simulink library "HardwareCommunication"  (R2016b)
settings: Solver=VariableStepAuto  StartTime=0.0  StopTime=10.0  RelTol=1e-3
undefined symbols (not defined in the file or in its folder): ReceiveFromInputDevice, SendToInputDevice
libraries: inSOMANET x8, SendToSOMANET x8, VariousLibrary x4, GESHandler x3, InputDeviceHandler x3, PDBHandler x3, SOMANETHandler x3, xpcethercatlib x2, ReceiveFromGES x2, ReceiveFromPDB x2, SendToPDB x2, InCommunication x1
settings Model: Creator=march  LastModifiedBy=march

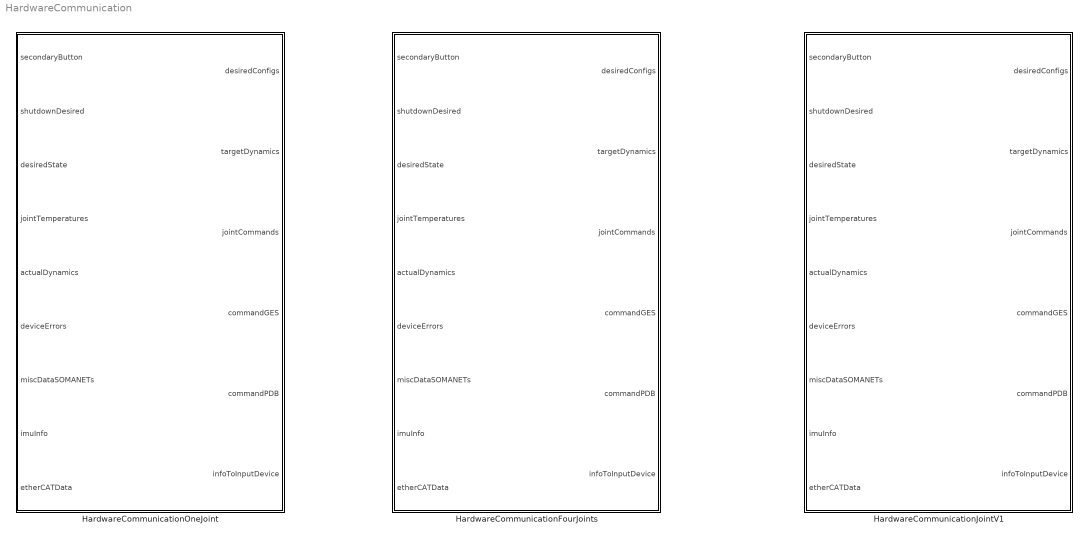
== system HardwareCommunication ==
  HardwareCommunicationFourJoints : Subsystem
  HardwareCommunicationJointV1 : Subsystem  AncestorBlock=HardwareCommunication/HardwareCommunicationOneJoint
  HardwareCommunicationOneJoint : Subsystem

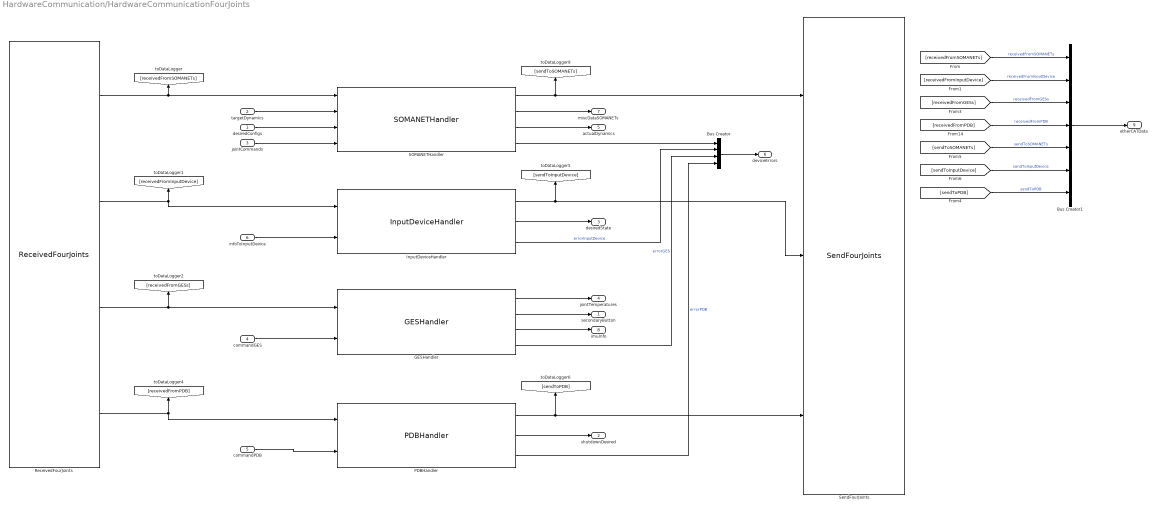
== system HardwareCommunication/HardwareCommunicationFourJoints ==
  desiredConfigs : Inport
  targetDynamics : Inport  Port=2
  jointCommands : Inport  Port=3
  commandGES : Inport  Port=4
  commandPDB : Inport  Port=5
  infoToInputDevice : Inport  Port=6
  Bus Creator : BusCreator  Inputs=4  OutDataTypeStr=Bus: DeviceErrors  NonVirtualBus=on
  Bus Creator1 : BusCreator  Inputs=7  OutDataTypeStr=Bus: EtherCATData  NonVirtualBus=on
  GESHandler : GESHandler/GESHandler
  InputDeviceHandler : InputDeviceHandler/InputDeviceHandler
  PDBHandler : PDBHandler/PDBHandler
  ReceivedFourJoints : InCommunication/ReceivedFourJoints
  SOMANETHandler : SOMANETHandler/SOMANETHandler
  SendFourJoints : OutCommunication/SendFourJoints
  secondaryButton : Outport
  shutdownDesired : Outport  Port=2
  desiredState : Outport  Port=3
  jointTemperatures : Outport  Port=4
  actualDynamics : Outport  Port=5
  deviceErrors : Outport  Port=6
  miscDataSOMANETs : Outport  Port=7
  imuInfo : Outport  Port=8
  etherCATData : Outport  Port=9
  wires:
  infoToInputDevice/1 -> InputDeviceHandler/2
  ReceivedFourJoints/3 -> GESHandler/1, [receivedFromGESs]
  ReceivedFourJoints/2 -> InputDeviceHandler/1, [receivedFromInputDevice]
  ReceivedFourJoints/4 -> PDBHandler/1, [receivedFromPDB]
  InputDeviceHandler/1 -> SendFourJoints/2, [sendToInputDevice]
  InputDeviceHandler/3 -> Bus Creator/2  "errorInputDevice"
  Bus Creator/1 -> deviceErrors/1
  PDBHandler/1 -> SendFourJoints/3, [sendToPDB]
  [receivedFromInputDevice] -> Bus Creator1/2  "receivedFromInputDevice"
  [receivedFromSOMANETs] -> Bus Creator1/1  "receivedFromSOMANETs"
  SOMANETHandler/2 -> miscDataSOMANETs/1
  [sendToPDB] -> Bus Creator1/7  "sendToPDB"
  ReceivedFourJoints/1 -> [receivedFromSOMANETs], SOMANETHandler/1
  GESHandler/2 -> secondaryButton/1
  SOMANETHandler/1 -> SendFourJoints/1, [sendToSOMANETs]
  InputDeviceHandler/2 -> desiredState/1
  jointCommands/1 -> SOMANETHandler/4
  SOMANETHandler/3 -> actualDynamics/1
  [sendToSOMANETs] -> Bus Creator1/5  "sendToSOMANETs"
  [sendToInputDevice] -> Bus Creator1/6  "sendToInputDevice"
  [receivedFromGESs] -> Bus Creator1/3  "receivedFromGESs"
  SOMANETHandler/4 -> Bus Creator/1
  desiredConfigs/1 -> SOMANETHandler/3
  [receivedFromPDB] -> Bus Creator1/4  "receivedFromPDB"
  Bus Creator1/1 -> etherCATData/1
  GESHandler/1 -> jointTemperatures/1
  PDBHandler/3 -> Bus Creator/4  "errorPDB"
  commandGES/1 -> GESHandler/2
  GESHandler/4 -> Bus Creator/3  "errorGES"
  commandPDB/1 -> PDBHandler/2
  PDBHandler/2 -> shutdownDesired/1
  targetDynamics/1 -> SOMANETHandler/2
  GESHandler/3 -> imuInfo/1

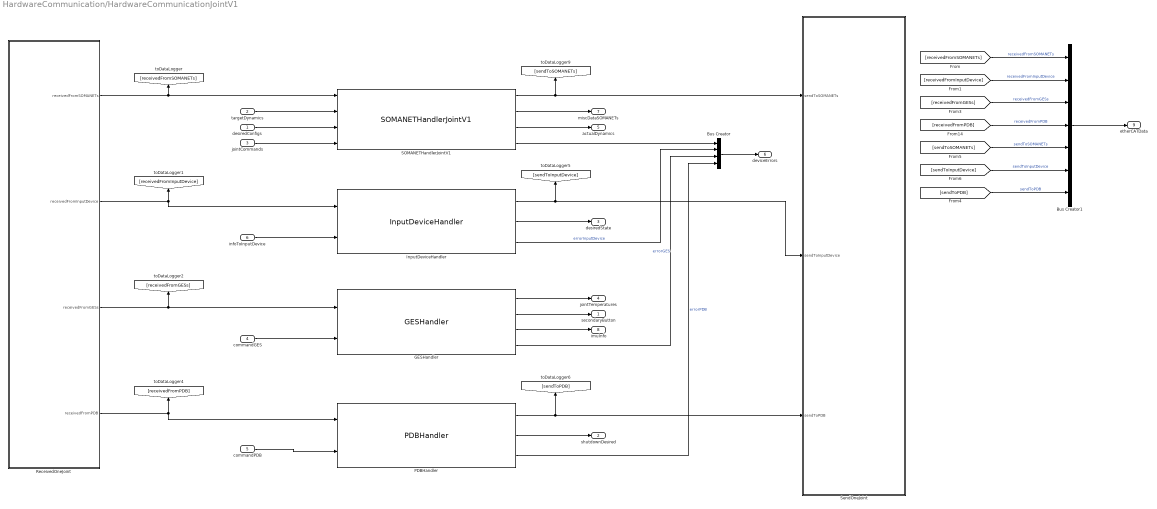
== system HardwareCommunication/HardwareCommunicationJointV1 ==
  desiredConfigs : Inport
  targetDynamics : Inport  Port=2
  jointCommands : Inport  Port=3
  commandGES : Inport  Port=4
  commandPDB : Inport  Port=5
  infoToInputDevice : Inport  Port=6
  Bus Creator : BusCreator  Inputs=4  OutDataTypeStr=Bus: DeviceErrors  NonVirtualBus=on
  Bus Creator1 : BusCreator  Inputs=7  OutDataTypeStr=Bus: EtherCATData  NonVirtualBus=on
  GESHandler : GESHandler/GESHandler
  InputDeviceHandler : InputDeviceHandler/InputDeviceHandler
  PDBHandler : PDBHandler/PDBHandler
  ReceivedOneJoint : Subsystem  AncestorBlock=InCommunication/ReceivedOneJoint
  SOMANETHandlerJointV1 : SOMANETHandler/SOMANETHandlerJointV1
  SendOneJoint : Subsystem  AncestorBlock=OutCommunication/SendOneJoint
  secondaryButton : Outport
  shutdownDesired : Outport  Port=2
  desiredState : Outport  Port=3
  jointTemperatures : Outport  Port=4
  actualDynamics : Outport  Port=5
  deviceErrors : Outport  Port=6
  miscDataSOMANETs : Outport  Port=7
  imuInfo : Outport  Port=8
  etherCATData : Outport  Port=9
  wires:
  infoToInputDevice/1 -> InputDeviceHandler/2
  ReceivedOneJoint/3(receivedFromGESs) -> GESHandler/1, [receivedFromGESs]
  ReceivedOneJoint/2(receivedFromInputDevice) -> InputDeviceHandler/1, [receivedFromInputDevice]
  ReceivedOneJoint/4(receivedFromPDB) -> PDBHandler/1, [receivedFromPDB]
  InputDeviceHandler/1 -> SendOneJoint/2(sendToInputDevice), [sendToInputDevice]
  InputDeviceHandler/3 -> Bus Creator/2  "errorInputDevice"
  Bus Creator/1 -> deviceErrors/1
  PDBHandler/1 -> SendOneJoint/3(sendToPDB), [sendToPDB]
  [receivedFromInputDevice] -> Bus Creator1/2  "receivedFromInputDevice"
  [receivedFromSOMANETs] -> Bus Creator1/1  "receivedFromSOMANETs"
  SOMANETHandlerJointV1/2 -> miscDataSOMANETs/1
  [sendToPDB] -> Bus Creator1/7  "sendToPDB"
  ReceivedOneJoint/1(receivedFromSOMANETs) -> SOMANETHandlerJointV1/1, [receivedFromSOMANETs]
  GESHandler/2 -> secondaryButton/1
  SOMANETHandlerJointV1/1 -> SendOneJoint/1(sendToSOMANETs), [sendToSOMANETs]
  InputDeviceHandler/2 -> desiredState/1
  jointCommands/1 -> SOMANETHandlerJointV1/4
  SOMANETHandlerJointV1/3 -> actualDynamics/1
  [sendToSOMANETs] -> Bus Creator1/5  "sendToSOMANETs"
  [sendToInputDevice] -> Bus Creator1/6  "sendToInputDevice"
  [receivedFromGESs] -> Bus Creator1/3  "receivedFromGESs"
  SOMANETHandlerJointV1/4 -> Bus Creator/1
  desiredConfigs/1 -> SOMANETHandlerJointV1/3
  [receivedFromPDB] -> Bus Creator1/4  "receivedFromPDB"
  Bus Creator1/1 -> etherCATData/1
  GESHandler/1 -> jointTemperatures/1
  PDBHandler/3 -> Bus Creator/4  "errorPDB"
  commandGES/1 -> GESHandler/2
  GESHandler/4 -> Bus Creator/3  "errorGES"
  commandPDB/1 -> PDBHandler/2
  PDBHandler/2 -> shutdownDesired/1
  targetDynamics/1 -> SOMANETHandlerJointV1/2
  GESHandler/3 -> imuInfo/1

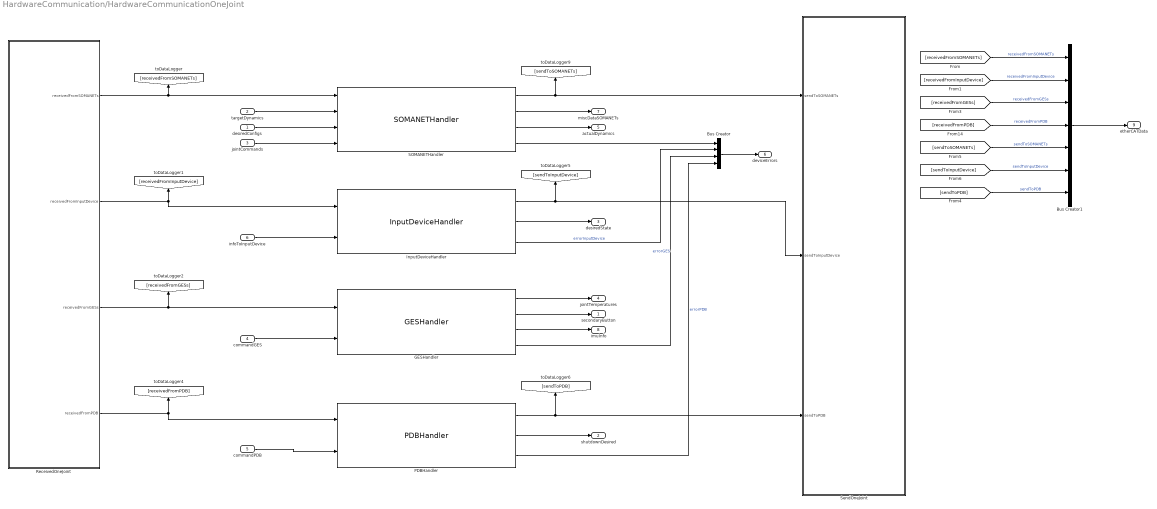
== system HardwareCommunication/HardwareCommunicationOneJoint ==
  desiredConfigs : Inport
  targetDynamics : Inport  Port=2
  jointCommands : Inport  Port=3
  commandGES : Inport  Port=4
  commandPDB : Inport  Port=5
  infoToInputDevice : Inport  Port=6
  Bus Creator : BusCreator  Inputs=4  OutDataTypeStr=Bus: DeviceErrors  NonVirtualBus=on
  Bus Creator1 : BusCreator  Inputs=7  OutDataTypeStr=Bus: EtherCATData  NonVirtualBus=on
  GESHandler : GESHandler/GESHandler
  InputDeviceHandler : InputDeviceHandler/InputDeviceHandler
  PDBHandler : PDBHandler/PDBHandler
  ReceivedOneJoint : Subsystem  AncestorBlock=InCommunication/ReceivedOneJoint
  SOMANETHandler : SOMANETHandler/SOMANETHandler
  SendOneJoint : Subsystem  AncestorBlock=OutCommunication/SendOneJoint
  secondaryButton : Outport
  shutdownDesired : Outport  Port=2
  desiredState : Outport  Port=3
  jointTemperatures : Outport  Port=4
  actualDynamics : Outport  Port=5
  deviceErrors : Outport  Port=6
  miscDataSOMANETs : Outport  Port=7
  imuInfo : Outport  Port=8
  etherCATData : Outport  Port=9
  wires:
  infoToInputDevice/1 -> InputDeviceHandler/2
  ReceivedOneJoint/3(receivedFromGESs) -> GESHandler/1, [receivedFromGESs]
  ReceivedOneJoint/2(receivedFromInputDevice) -> InputDeviceHandler/1, [receivedFromInputDevice]
  ReceivedOneJoint/4(receivedFromPDB) -> PDBHandler/1, [receivedFromPDB]
  InputDeviceHandler/1 -> SendOneJoint/2(sendToInputDevice), [sendToInputDevice]
  InputDeviceHandler/3 -> Bus Creator/2  "errorInputDevice"
  Bus Creator/1 -> deviceErrors/1
  PDBHandler/1 -> SendOneJoint/3(sendToPDB), [sendToPDB]
  [receivedFromInputDevice] -> Bus Creator1/2  "receivedFromInputDevice"
  [receivedFromSOMANETs] -> Bus Creator1/1  "receivedFromSOMANETs"
  SOMANETHandler/2 -> miscDataSOMANETs/1
  [sendToPDB] -> Bus Creator1/7  "sendToPDB"
  ReceivedOneJoint/1(receivedFromSOMANETs) -> [receivedFromSOMANETs], SOMANETHandler/1
  GESHandler/2 -> secondaryButton/1
  SOMANETHandler/1 -> SendOneJoint/1(sendToSOMANETs), [sendToSOMANETs]
  InputDeviceHandler/2 -> desiredState/1
  jointCommands/1 -> SOMANETHandler/4
  SOMANETHandler/3 -> actualDynamics/1
  [sendToSOMANETs] -> Bus Creator1/5  "sendToSOMANETs"
  [sendToInputDevice] -> Bus Creator1/6  "sendToInputDevice"
  [receivedFromGESs] -> Bus Creator1/3  "receivedFromGESs"
  SOMANETHandler/4 -> Bus Creator/1
  desiredConfigs/1 -> SOMANETHandler/3
  [receivedFromPDB] -> Bus Creator1/4  "receivedFromPDB"
  Bus Creator1/1 -> etherCATData/1
  GESHandler/1 -> jointTemperatures/1
  PDBHandler/3 -> Bus Creator/4  "errorPDB"
  commandGES/1 -> GESHandler/2
  GESHandler/4 -> Bus Creator/3  "errorGES"
  commandPDB/1 -> PDBHandler/2
  PDBHandler/2 -> shutdownDesired/1
  targetDynamics/1 -> SOMANETHandler/2
  GESHandler/3 -> imuInfo/1

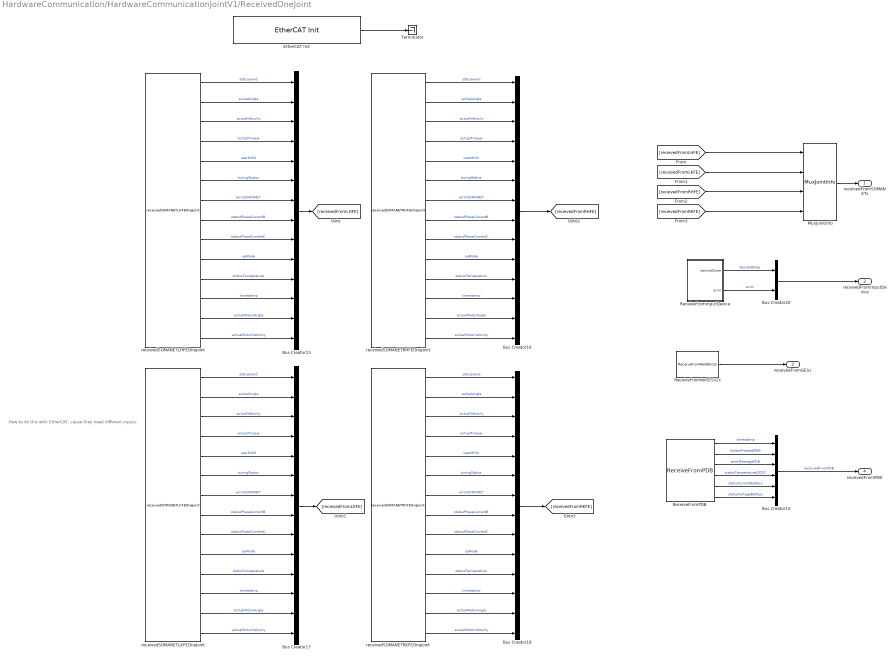
== system HardwareCommunication/HardwareCommunicationJointV1/ReceivedOneJoint ==
  note: How to do this with EtherCAT, cause they need different inputs.
  Bus Creator10 : BusCreator  Inputs=6  OutDataTypeStr=Bus: EtherCATReceivedFromPDB  NonVirtualBus=on
  Bus Creator{15..18} (4 alike) : BusCreator  Inputs=14  OutDataTypeStr=Bus: EtherCATReceivedFromSOMANET  NonVirtualBus=on
  Bus Creator20 : BusCreator  Inputs=2  OutDataTypeStr=Bus: EtherCATReceivedFromInputDevice  NonVirtualBus=on
  "EtherCAT Init " : xpcethercatlib/EtherCAT Init   Priority=0  config_file=..\EcatXML\SingleJointNoGES_eni.xml  device_id=0  pci_bus=2  pci_slot=0  dctuning=0  enaDebug=off  enaDC=on  errLink=on  masterDbg=on  stateChgDbg=on  baseClock=off  masterCfg=off  logFile='c:\dbglog.txt'  sample_time=0.002000  DCMode=0
  MuxJointInfo : VariousLibrary/MuxJointInfo
  ReceiveFromInputDevice : Subsystem  AncestorBlock=ReceiveFromInputDevice/ReceiveFromInputDevice
  ReceiveFromNoGESv2s : ReceiveFromGES/ReceiveFromNoGESv2s
  ReceiveFromPDB : ReceiveFromPDB/ReceiveFromPDB
  Terminator : Terminator
  receivedSOMANETLHFEOneJoint : inSOMANET/receivedSOMANETLHFEOneJoint
  receivedSOMANETLKFEOneJoint : inSOMANET/receivedSOMANETLKFEOneJoint
  receivedSOMANETRHFEOneJoint : inSOMANET/receivedSOMANETRHFEOneJoint
  receivedSOMANETRKFEOneJoint : inSOMANET/receivedSOMANETRKFEOneJoint
  receivedFromSOMANETs : Outport  OutDataTypeStr=Bus: EtherCATReceivedFromSOMANET  PortDimensions=[ 1 4 ]  BusOutputAsStruct=on
  receivedFromInputDevice : Outport  Port=2  OutDataTypeStr=Bus: EtherCATReceivedFromInputDevice  BusOutputAsStruct=on
  receivedFromGESs : Outport  Port=3  OutDataTypeStr=Bus: EtherCATReceivedFromGES  PortDimensions=[1 3]  BusOutputAsStruct=on
  receivedFromPDB : Outport  Port=4  OutDataTypeStr=Bus: EtherCATReceivedFromPDB  BusOutputAsStruct=on
  wires:
  ReceiveFromPDB/1 -> Bus Creator10/1  "timestamp"
  ReceiveFromPDB/6 -> Bus Creator10/6  "statusVoltageBattery"
  ReceiveFromPDB/5 -> Bus Creator10/5  "statusCurrentBattery"
  ReceiveFromPDB/4 -> Bus Creator10/4  "statusTemperatureDCDC"
  ReceiveFromPDB/3 -> Bus Creator10/3  "errorMessagePDB"
  ReceiveFromPDB/2 -> Bus Creator10/2  "buttonPressedPDB"
  [receivedFromLKFE] -> MuxJointInfo/2
  [receivedFromRKFE] -> MuxJointInfo/4
  [receivedFromRHFE] -> MuxJointInfo/3
  [receivedFromLHFE] -> MuxJointInfo/1
  Bus Creator20/1 -> receivedFromInputDevice/1
  ReceiveFromInputDevice/2(error) -> Bus Creator20/2  "error"
  Bus Creator18/1 -> [receivedFromRKFE]
  receivedSOMANETRKFEOneJoint/11 -> Bus Creator18/11  "statusTemperature"
  receivedSOMANETLKFEOneJoint/11 -> Bus Creator17/11  "statusTemperature"
  receivedSOMANETRKFEOneJoint/12 -> Bus Creator18/12  "timestamp"
  receivedSOMANETRKFEOneJoint/6 -> Bus Creator18/6  "tuningStatus"
  receivedSOMANETRKFEOneJoint/1 -> Bus Creator18/1  "statusword"
  receivedSOMANETLKFEOneJoint/5 -> Bus Creator17/5  "userMISO"
  receivedSOMANETRKFEOneJoint/7 -> Bus Creator18/7  "errorSOMANET"
  receivedSOMANETRKFEOneJoint/8 -> Bus Creator18/8  "statusPhaseCurrentB"
  receivedSOMANETRKFEOneJoint/3 -> Bus Creator18/3  "actualVelocity"
  receivedSOMANETRKFEOneJoint/5 -> Bus Creator18/5  "userMISO"
  receivedSOMANETLKFEOneJoint/8 -> Bus Creator17/8  "statusPhaseCurrentB"
  receivedSOMANETLKFEOneJoint/12 -> Bus Creator17/12  "timestamp"
  Bus Creator17/1 -> [receivedFromLKFE]
  receivedSOMANETRKFEOneJoint/10 -> Bus Creator18/10  "opMode"
  receivedSOMANETLKFEOneJoint/6 -> Bus Creator17/6  "tuningStatus"
  ReceiveFromInputDevice/1(desiredState) -> Bus Creator20/1  "desiredState"
  receivedSOMANETLKFEOneJoint/10 -> Bus Creator17/10  "opMode"
  receivedSOMANETRKFEOneJoint/2 -> Bus Creator18/2  "actualAngle"
  receivedSOMANETRKFEOneJoint/9 -> Bus Creator18/9  "statusPhaseCurrentC"
  receivedSOMANETRKFEOneJoint/4 -> Bus Creator18/4  "actualTorque"
  receivedSOMANETLKFEOneJoint/9 -> Bus Creator17/9  "statusPhaseCurrentC"
  receivedSOMANETLHFEOneJoint/9 -> Bus Creator15/9  "statusPhaseCurrentC"
  receivedSOMANETLKFEOneJoint/7 -> Bus Creator17/7  "errorSOMANET"
  receivedSOMANETLKFEOneJoint/4 -> Bus Creator17/4  "actualTorque"
  MuxJointInfo/1 -> receivedFromSOMANETs/1
  receivedSOMANETLKFEOneJoint/3 -> Bus Creator17/3  "actualVelocity"
  receivedSOMANETRHFEOneJoint/8 -> Bus Creator16/8  "statusPhaseCurrentB"
  receivedSOMANETRHFEOneJoint/5 -> Bus Creator16/5  "userMISO"
  receivedSOMANETLHFEOneJoint/8 -> Bus Creator15/8  "statusPhaseCurrentB"
  receivedSOMANETLHFEOneJoint/4 -> Bus Creator15/4  "actualTorque"
  receivedSOMANETLHFEOneJoint/12 -> Bus Creator15/12  "timestamp"
  receivedSOMANETLKFEOneJoint/2 -> Bus Creator17/2  "actualAngle"
  receivedSOMANETRHFEOneJoint/12 -> Bus Creator16/12  "timestamp"
  receivedSOMANETLHFEOneJoint/3 -> Bus Creator15/3  "actualVelocity"
  receivedSOMANETLKFEOneJoint/1 -> Bus Creator17/1  "statusword"
  Bus Creator16/1 -> [receivedFromRHFE]
  Bus Creator15/1 -> [receivedFromLHFE]
  receivedSOMANETRHFEOneJoint/11 -> Bus Creator16/11  "statusTemperature"
  receivedSOMANETLHFEOneJoint/7 -> Bus Creator15/7  "errorSOMANET"
  receivedSOMANETRHFEOneJoint/10 -> Bus Creator16/10  "opMode"
  receivedSOMANETRHFEOneJoint/9 -> Bus Creator16/9  "statusPhaseCurrentC"
  receivedSOMANETRHFEOneJoint/7 -> Bus Creator16/7  "errorSOMANET"
  receivedSOMANETRHFEOneJoint/1 -> Bus Creator16/1  "statusword"
  receivedSOMANETLHFEOneJoint/2 -> Bus Creator15/2  "actualAngle"
  receivedSOMANETRHFEOneJoint/6 -> Bus Creator16/6  "tuningStatus"
  receivedSOMANETRHFEOneJoint/4 -> Bus Creator16/4  "actualTorque"
  receivedSOMANETRHFEOneJoint/3 -> Bus Creator16/3  "actualVelocity"
  receivedSOMANETRHFEOneJoint/2 -> Bus Creator16/2  "actualAngle"
  receivedSOMANETLHFEOneJoint/11 -> Bus Creator15/11  "statusTemperature"
  receivedSOMANETLHFEOneJoint/1 -> Bus Creator15/1  "statusword"
  receivedSOMANETLHFEOneJoint/10 -> Bus Creator15/10  "opMode"
  receivedSOMANETLHFEOneJoint/6 -> Bus Creator15/6  "tuningStatus"
  Bus Creator10/1 -> receivedFromPDB/1  "receivedFromPDB"
  receivedSOMANETLHFEOneJoint/5 -> Bus Creator15/5  "userMISO"
  "EtherCAT Init "/1 -> Terminator/1
  receivedSOMANETLHFEOneJoint/13 -> Bus Creator15/13  "actualMotorAngle"
  receivedSOMANETLHFEOneJoint/14 -> Bus Creator15/14  "actualMotorVelocity"
  receivedSOMANETLKFEOneJoint/13 -> Bus Creator17/13  "actualMotorAngle"
  receivedSOMANETLKFEOneJoint/14 -> Bus Creator17/14  "actualMotorVelocity"
  receivedSOMANETRKFEOneJoint/13 -> Bus Creator18/13  "actualMotorAngle"
  receivedSOMANETRKFEOneJoint/14 -> Bus Creator18/14  "actualMotorVelocity"
  receivedSOMANETRHFEOneJoint/13 -> Bus Creator16/13  "actualMotorAngle"
  receivedSOMANETRHFEOneJoint/14 -> Bus Creator16/14  "actualMotorVelocity"
  ReceiveFromNoGESv2s/1 -> receivedFromGESs/1

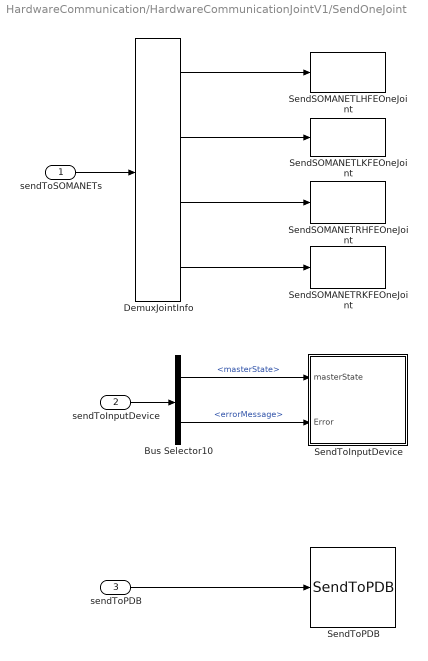
== system HardwareCommunication/HardwareCommunicationJointV1/SendOneJoint ==
  sendToSOMANETs : Inport  OutDataTypeStr=Bus: EtherCATSendToSOMANET  PortDimensions=[1 4]  BusOutputAsStruct=on
  sendToInputDevice : Inport  Port=2  OutDataTypeStr=Bus: EtherCATSendToInputDevice  BusOutputAsStruct=on
  sendToPDB : Inport  Port=3  OutDataTypeStr=Bus: EtherCATSendToPDB  BusOutputAsStruct=on
  Bus Selector10 : BusSelector  OutputSignals=masterState,errorMessage
  DemuxJointInfo : VariousLibrary/DemuxJointInfo
  SendSOMANETLHFEOneJoint : SendToSOMANET/SendSOMANETLHFEOneJoint
  SendSOMANETLKFEOneJoint : SendToSOMANET/SendSOMANETLKFEOneJoint
  SendSOMANETRHFEOneJoint : SendToSOMANET/SendSOMANETRHFEOneJoint
  SendSOMANETRKFEOneJoint : SendToSOMANET/SendSOMANETRKFEOneJoint
  SendToInputDevice : Subsystem  AncestorBlock=SendToInputDevice/SendToInputDevice
  SendToPDB : SendToPDB/SendToPDB
  wires:
  sendToInputDevice/1 -> Bus Selector10/1
  DemuxJointInfo/4 -> SendSOMANETRKFEOneJoint/1
  Bus Selector10/1 -> SendToInputDevice/1(masterState)  "<masterState>"
  sendToPDB/1 -> SendToPDB/1
  Bus Selector10/2 -> SendToInputDevice/2(Error)  "<errorMessage>"
  DemuxJointInfo/1 -> SendSOMANETLHFEOneJoint/1
  DemuxJointInfo/2 -> SendSOMANETLKFEOneJoint/1
  DemuxJointInfo/3 -> SendSOMANETRHFEOneJoint/1
  sendToSOMANETs/1 -> DemuxJointInfo/1

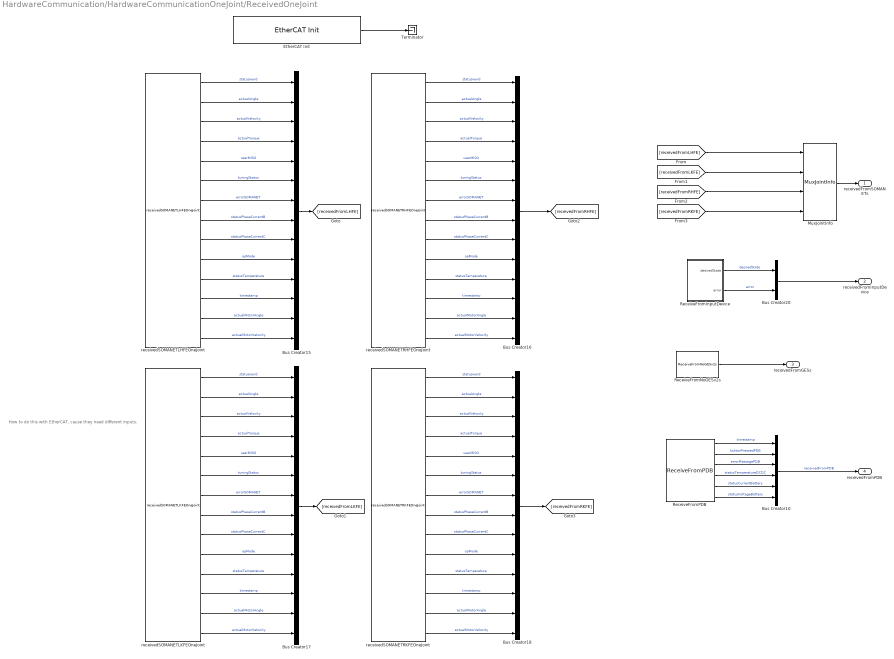
== system HardwareCommunication/HardwareCommunicationOneJoint/ReceivedOneJoint ==
  note: How to do this with EtherCAT, cause they need different inputs.
  Bus Creator10 : BusCreator  Inputs=6  OutDataTypeStr=Bus: EtherCATReceivedFromPDB  NonVirtualBus=on
  Bus Creator{15..18} (4 alike) : BusCreator  Inputs=14  OutDataTypeStr=Bus: EtherCATReceivedFromSOMANET  NonVirtualBus=on
  Bus Creator20 : BusCreator  Inputs=2  OutDataTypeStr=Bus: EtherCATReceivedFromInputDevice  NonVirtualBus=on
  "EtherCAT Init " : xpcethercatlib/EtherCAT Init   Priority=0  config_file=..\EcatXML\SingleJointNoGES_eni.xml  device_id=0  pci_bus=2  pci_slot=0  dctuning=0  enaDebug=off  enaDC=on  errLink=on  masterDbg=on  stateChgDbg=on  baseClock=off  masterCfg=off  logFile='c:\dbglog.txt'  sample_time=0.002000  DCMode=0
  MuxJointInfo : VariousLibrary/MuxJointInfo
  ReceiveFromInputDevice : Subsystem  AncestorBlock=ReceiveFromInputDevice/ReceiveFromInputDevice
  ReceiveFromNoGESv2s : ReceiveFromGES/ReceiveFromNoGESv2s
  ReceiveFromPDB : ReceiveFromPDB/ReceiveFromPDB
  Terminator : Terminator
  receivedSOMANETLHFEOneJoint : inSOMANET/receivedSOMANETLHFEOneJoint
  receivedSOMANETLKFEOneJoint : inSOMANET/receivedSOMANETLKFEOneJoint
  receivedSOMANETRHFEOneJoint : inSOMANET/receivedSOMANETRHFEOneJoint
  receivedSOMANETRKFEOneJoint : inSOMANET/receivedSOMANETRKFEOneJoint
  receivedFromSOMANETs : Outport  OutDataTypeStr=Bus: EtherCATReceivedFromSOMANET  PortDimensions=[ 1 4 ]  BusOutputAsStruct=on
  receivedFromInputDevice : Outport  Port=2  OutDataTypeStr=Bus: EtherCATReceivedFromInputDevice  BusOutputAsStruct=on
  receivedFromGESs : Outport  Port=3  OutDataTypeStr=Bus: EtherCATReceivedFromGES  PortDimensions=[1 3]  BusOutputAsStruct=on
  receivedFromPDB : Outport  Port=4  OutDataTypeStr=Bus: EtherCATReceivedFromPDB  BusOutputAsStruct=on
  wires:
  ReceiveFromPDB/1 -> Bus Creator10/1  "timestamp"
  ReceiveFromPDB/6 -> Bus Creator10/6  "statusVoltageBattery"
  ReceiveFromPDB/5 -> Bus Creator10/5  "statusCurrentBattery"
  ReceiveFromPDB/4 -> Bus Creator10/4  "statusTemperatureDCDC"
  ReceiveFromPDB/3 -> Bus Creator10/3  "errorMessagePDB"
  ReceiveFromPDB/2 -> Bus Creator10/2  "buttonPressedPDB"
  [receivedFromLKFE] -> MuxJointInfo/2
  [receivedFromRKFE] -> MuxJointInfo/4
  [receivedFromRHFE] -> MuxJointInfo/3
  [receivedFromLHFE] -> MuxJointInfo/1
  Bus Creator20/1 -> receivedFromInputDevice/1
  ReceiveFromInputDevice/2(error) -> Bus Creator20/2  "error"
  Bus Creator18/1 -> [receivedFromRKFE]
  receivedSOMANETRKFEOneJoint/11 -> Bus Creator18/11  "statusTemperature"
  receivedSOMANETLKFEOneJoint/11 -> Bus Creator17/11  "statusTemperature"
  receivedSOMANETRKFEOneJoint/12 -> Bus Creator18/12  "timestamp"
  receivedSOMANETRKFEOneJoint/6 -> Bus Creator18/6  "tuningStatus"
  receivedSOMANETRKFEOneJoint/1 -> Bus Creator18/1  "statusword"
  receivedSOMANETLKFEOneJoint/5 -> Bus Creator17/5  "userMISO"
  receivedSOMANETRKFEOneJoint/7 -> Bus Creator18/7  "errorSOMANET"
  receivedSOMANETRKFEOneJoint/8 -> Bus Creator18/8  "statusPhaseCurrentB"
  receivedSOMANETRKFEOneJoint/3 -> Bus Creator18/3  "actualVelocity"
  receivedSOMANETRKFEOneJoint/5 -> Bus Creator18/5  "userMISO"
  receivedSOMANETLKFEOneJoint/8 -> Bus Creator17/8  "statusPhaseCurrentB"
  receivedSOMANETLKFEOneJoint/12 -> Bus Creator17/12  "timestamp"
  Bus Creator17/1 -> [receivedFromLKFE]
  receivedSOMANETRKFEOneJoint/10 -> Bus Creator18/10  "opMode"
  receivedSOMANETLKFEOneJoint/6 -> Bus Creator17/6  "tuningStatus"
  ReceiveFromInputDevice/1(desiredState) -> Bus Creator20/1  "desiredState"
  receivedSOMANETLKFEOneJoint/10 -> Bus Creator17/10  "opMode"
  receivedSOMANETRKFEOneJoint/2 -> Bus Creator18/2  "actualAngle"
  receivedSOMANETRKFEOneJoint/9 -> Bus Creator18/9  "statusPhaseCurrentC"
  receivedSOMANETRKFEOneJoint/4 -> Bus Creator18/4  "actualTorque"
  receivedSOMANETLKFEOneJoint/9 -> Bus Creator17/9  "statusPhaseCurrentC"
  receivedSOMANETLHFEOneJoint/9 -> Bus Creator15/9  "statusPhaseCurrentC"
  receivedSOMANETLKFEOneJoint/7 -> Bus Creator17/7  "errorSOMANET"
  receivedSOMANETLKFEOneJoint/4 -> Bus Creator17/4  "actualTorque"
  MuxJointInfo/1 -> receivedFromSOMANETs/1
  receivedSOMANETLKFEOneJoint/3 -> Bus Creator17/3  "actualVelocity"
  receivedSOMANETRHFEOneJoint/8 -> Bus Creator16/8  "statusPhaseCurrentB"
  receivedSOMANETRHFEOneJoint/5 -> Bus Creator16/5  "userMISO"
  receivedSOMANETLHFEOneJoint/8 -> Bus Creator15/8  "statusPhaseCurrentB"
  receivedSOMANETLHFEOneJoint/4 -> Bus Creator15/4  "actualTorque"
  receivedSOMANETLHFEOneJoint/12 -> Bus Creator15/12  "timestamp"
  receivedSOMANETLKFEOneJoint/2 -> Bus Creator17/2  "actualAngle"
  receivedSOMANETRHFEOneJoint/12 -> Bus Creator16/12  "timestamp"
  receivedSOMANETLHFEOneJoint/3 -> Bus Creator15/3  "actualVelocity"
  receivedSOMANETLKFEOneJoint/1 -> Bus Creator17/1  "statusword"
  Bus Creator16/1 -> [receivedFromRHFE]
  Bus Creator15/1 -> [receivedFromLHFE]
  receivedSOMANETRHFEOneJoint/11 -> Bus Creator16/11  "statusTemperature"
  receivedSOMANETLHFEOneJoint/7 -> Bus Creator15/7  "errorSOMANET"
  receivedSOMANETRHFEOneJoint/10 -> Bus Creator16/10  "opMode"
  receivedSOMANETRHFEOneJoint/9 -> Bus Creator16/9  "statusPhaseCurrentC"
  receivedSOMANETRHFEOneJoint/7 -> Bus Creator16/7  "errorSOMANET"
  receivedSOMANETRHFEOneJoint/1 -> Bus Creator16/1  "statusword"
  receivedSOMANETLHFEOneJoint/2 -> Bus Creator15/2  "actualAngle"
  receivedSOMANETRHFEOneJoint/6 -> Bus Creator16/6  "tuningStatus"
  receivedSOMANETRHFEOneJoint/4 -> Bus Creator16/4  "actualTorque"
  receivedSOMANETRHFEOneJoint/3 -> Bus Creator16/3  "actualVelocity"
  receivedSOMANETRHFEOneJoint/2 -> Bus Creator16/2  "actualAngle"
  receivedSOMANETLHFEOneJoint/11 -> Bus Creator15/11  "statusTemperature"
  receivedSOMANETLHFEOneJoint/1 -> Bus Creator15/1  "statusword"
  receivedSOMANETLHFEOneJoint/10 -> Bus Creator15/10  "opMode"
  receivedSOMANETLHFEOneJoint/6 -> Bus Creator15/6  "tuningStatus"
  Bus Creator10/1 -> receivedFromPDB/1  "receivedFromPDB"
  receivedSOMANETLHFEOneJoint/5 -> Bus Creator15/5  "userMISO"
  "EtherCAT Init "/1 -> Terminator/1
  receivedSOMANETLHFEOneJoint/13 -> Bus Creator15/13  "actualMotorAngle"
  receivedSOMANETLHFEOneJoint/14 -> Bus Creator15/14  "actualMotorVelocity"
  receivedSOMANETLKFEOneJoint/13 -> Bus Creator17/13  "actualMotorAngle"
  receivedSOMANETLKFEOneJoint/14 -> Bus Creator17/14  "actualMotorVelocity"
  receivedSOMANETRKFEOneJoint/13 -> Bus Creator18/13  "actualMotorAngle"
  receivedSOMANETRKFEOneJoint/14 -> Bus Creator18/14  "actualMotorVelocity"
  receivedSOMANETRHFEOneJoint/13 -> Bus Creator16/13  "actualMotorAngle"
  receivedSOMANETRHFEOneJoint/14 -> Bus Creator16/14  "actualMotorVelocity"
  ReceiveFromNoGESv2s/1 -> receivedFromGESs/1

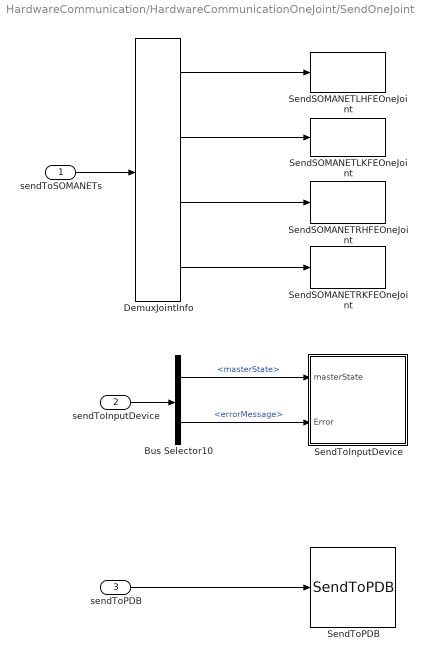
== system HardwareCommunication/HardwareCommunicationOneJoint/SendOneJoint ==
  sendToSOMANETs : Inport  OutDataTypeStr=Bus: EtherCATSendToSOMANET  PortDimensions=[1 4]  BusOutputAsStruct=on
  sendToInputDevice : Inport  Port=2  OutDataTypeStr=Bus: EtherCATSendToInputDevice  BusOutputAsStruct=on
  sendToPDB : Inport  Port=3  OutDataTypeStr=Bus: EtherCATSendToPDB  BusOutputAsStruct=on
  Bus Selector10 : BusSelector  OutputSignals=masterState,errorMessage
  DemuxJointInfo : VariousLibrary/DemuxJointInfo
  SendSOMANETLHFEOneJoint : SendToSOMANET/SendSOMANETLHFEOneJoint
  SendSOMANETLKFEOneJoint : SendToSOMANET/SendSOMANETLKFEOneJoint
  SendSOMANETRHFEOneJoint : SendToSOMANET/SendSOMANETRHFEOneJoint
  SendSOMANETRKFEOneJoint : SendToSOMANET/SendSOMANETRKFEOneJoint
  SendToInputDevice : Subsystem  AncestorBlock=SendToInputDevice/SendToInputDevice
  SendToPDB : SendToPDB/SendToPDB
  wires:
  sendToInputDevice/1 -> Bus Selector10/1
  DemuxJointInfo/4 -> SendSOMANETRKFEOneJoint/1
  Bus Selector10/1 -> SendToInputDevice/1(masterState)  "<masterState>"
  sendToPDB/1 -> SendToPDB/1
  Bus Selector10/2 -> SendToInputDevice/2(Error)  "<errorMessage>"
  DemuxJointInfo/1 -> SendSOMANETLHFEOneJoint/1
  DemuxJointInfo/2 -> SendSOMANETLKFEOneJoint/1
  DemuxJointInfo/3 -> SendSOMANETRHFEOneJoint/1
  sendToSOMANETs/1 -> DemuxJointInfo/1

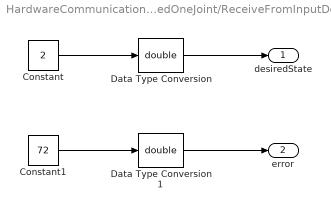
== system HardwareCommunication/HardwareCommunicationJointV1/ReceivedOneJoint/ReceiveFromInputDevice ==
  Constant : Constant  Value=2
  Constant1 : Constant  Value=72
  Data Type Conversion : DataTypeConversion  OutDataTypeStr=double
  Data Type Conversion1 : DataTypeConversion  OutDataTypeStr=double
  desiredState : Outport
  error : Outport  Port=2
  wires:
  Data Type Conversion/1 -> desiredState/1
  Data Type Conversion1/1 -> error/1
  Constant/1 -> Data Type Conversion/1
  Constant1/1 -> Data Type Conversion1/1

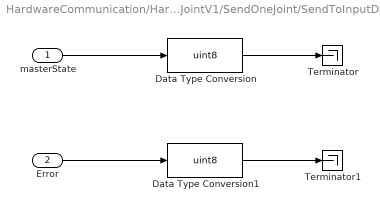
== system HardwareCommunication/HardwareCommunicationJointV1/SendOneJoint/SendToInputDevice ==
  masterState : Inport
  Error : Inport  Port=2
  Data Type Conversion : DataTypeConversion  OutDataTypeStr=uint8  RndMeth=Nearest
  Data Type Conversion1 : DataTypeConversion  OutDataTypeStr=uint8  RndMeth=Nearest
  Terminator : Terminator
  Terminator1 : Terminator
  wires:
  masterState/1 -> Data Type Conversion/1
  Error/1 -> Data Type Conversion1/1
  Data Type Conversion/1 -> Terminator/1
  Data Type Conversion1/1 -> Terminator1/1

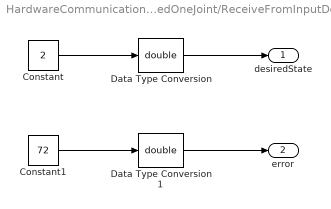
== system HardwareCommunication/HardwareCommunicationOneJoint/ReceivedOneJoint/ReceiveFromInputDevice ==
  Constant : Constant  Value=2
  Constant1 : Constant  Value=72
  Data Type Conversion : DataTypeConversion  OutDataTypeStr=double
  Data Type Conversion1 : DataTypeConversion  OutDataTypeStr=double
  desiredState : Outport
  error : Outport  Port=2
  wires:
  Data Type Conversion/1 -> desiredState/1
  Data Type Conversion1/1 -> error/1
  Constant/1 -> Data Type Conversion/1
  Constant1/1 -> Data Type Conversion1/1

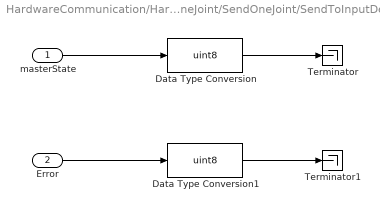
== system HardwareCommunication/HardwareCommunicationOneJoint/SendOneJoint/SendToInputDevice ==
  masterState : Inport
  Error : Inport  Port=2
  Data Type Conversion : DataTypeConversion  OutDataTypeStr=uint8  RndMeth=Nearest
  Data Type Conversion1 : DataTypeConversion  OutDataTypeStr=uint8  RndMeth=Nearest
  Terminator : Terminator
  Terminator1 : Terminator
  wires:
  masterState/1 -> Data Type Conversion/1
  Error/1 -> Data Type Conversion1/1
  Data Type Conversion/1 -> Terminator/1
  Data Type Conversion1/1 -> Terminator1/1
